simulink model "allelectronicsdraft"  (R2020a)
settings: Solver=VariableStepAuto  StartTime=0.0  StopTime=5  RelTol=1e-3
undefined symbols (not defined in the file): Ion, Lithium, sigbuilder_block
libraries: powerlib x15, electricdrivelib x13, powerlib_meascontrol x4, simulink x2, re_lib x1
settings Model: Creator=ASUS  LastModifiedBy=ASUS

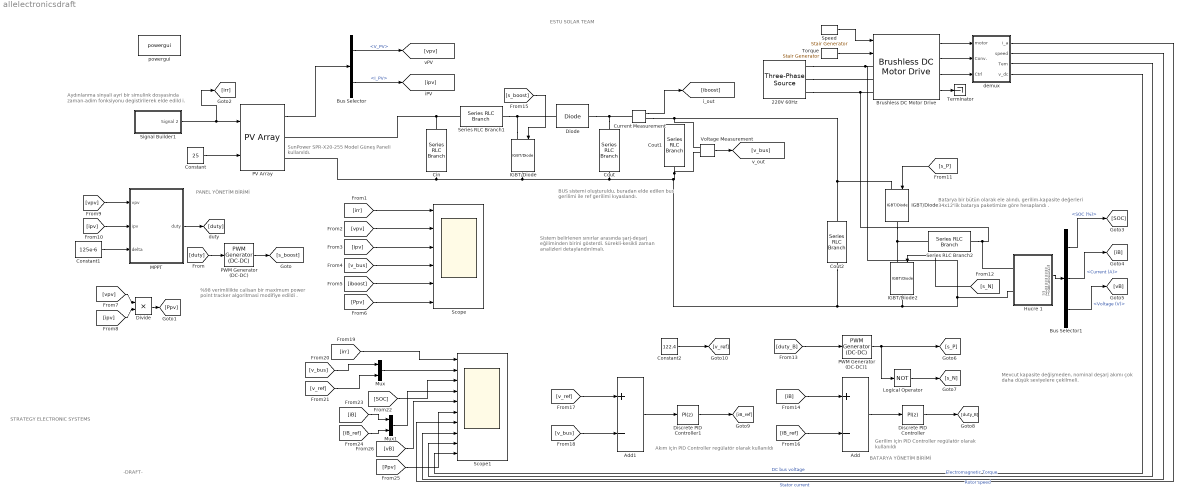
== system allelectronicsdraft ==
  note: -DRAFT-
  note: STRATEGY
      | ELECTRONIC SYSTEMS
  note: ESTU SOLAR TEAM
  note: Akım için PID Controller regülatör olarak kullanıldı
  note: PANEL YÖNETİM BİRİMİ
  note: BATARYA YÖNETİM BİRİMİ
  note: Gerilim için PID Controller regülatör olarak kullanıldı
  note: Aydınlanma sinyali ayri bir simulink dosyasinda
      | zaman-adim fonksiyonu degistirilerek elde edild i.
  note: %98 verimlilikte calisan bir maximum power
      | point tracker algoritmasi modifiye edildi .
  note: BUS sistemi oluşturuldu, buradan elde edilen
      | bus gerilimi ile ref gerilimi kıyaslandı.
  note: Batarya bir bütün olarak ele alındı, gerilim-kapasite değerleri
      | 34x12'lik batarya paketimize göre hesaplandı .
  note: Sistem belirlenen sınırlar arasında şarj-deşarj
      | eğiliminden birini gösterdi. Sürekli-kesikli zaman
      | analizleri detaylandırılmalı.
  note: Mevcut kapasite değişmeden, nominal deşarj akımı çok
      | daha düşük seviyelere çekilmeli.
  note: SunPower SPR-X20-255 Model Güneş Paneli kullanıldı.
  220V 60Hz : powerlib/Electrical Sources/Three-Phase Source  InternalConnection=Yg  VoltagePhases=off  Voltage=220  PhaseAngle=0  Voltage_phases=[25e3 25e3 25e3]/sqrt(3)  PhaseAngles_phases=[0 -120 +120]  Frequency=60  NonIdealSource=on  SpecifyImpedance=off  Resistance=0.02  Inductance=0.05e-3  ShortCircuitLevel=100e6  BaseVoltage=25e3  XRratio=7  BusType=swing  Pref=0  Qref=0  Prefabc=[10e3, 10e3, 10e3]  Qrefabc=[0, 0, 0]  Qmin=-inf  Qmax=inf
      settings: SourceProductBaseCode=MT,PS
  Add : Sum  Inputs=+-
  Add1 : Sum  Inputs=+-
  Brushless DC Motor Drive : electricdrivelib/AC drives/Brushless DC Motor Drive  Rs=0.2  Lls=8.5e-3  Flat=120  MachineConstant=Flux linkage established by magnets (V.s)  FluxCst=0.175  VoltageCst=146.6077  TorqueCst=1.4  ia=0  ib=0  J=0.089  Friction=0.005  p=4  wm=0  thetam=0  Rsnb_rec=10e3  Csnb_rec=20e-9  Ron_rec=1e-3  Vf_rec=1.3  cap_bus=2000e-6  Rbrake=8  fbrake=4000  activationVoltage=320  shutdownVoltage=310  deviceType=IGBT / Diodes  Ron_inv=1e-3  Vf_inv=0.8  Vfd_inv=0.8  Tf=1e-6  Tt=2e-6  Tf_GTO=10e-6  Tt_GTO=20e-6  Rsnb_inv=5000  Csnb_inv=inf  regulationType=Speed regulation  Acc=1000  Dec=-1000  kp_sc=3.3  ki_sc=300  fc_sc=285  Tsc=140e-6  Tmin=-17.8  Tmax=17.8  h=0.01  freq_max=20e3  Tvect=20e-6  zeta=0.99  Trd=0.13/5  K1=3000  K2=-49500  baseSampleTime=2e-06  outputBusMode=Multiple output buses  busLabels=off  sensorless=off  MechanicalLoad=Torque Tm  modelDetailLevel=Detailed  driveType=AC7  AverageValue=off
      settings: SourceProductBaseCode=PS
  Bus Selector : BusSelector  OutputSignals=V_PV,I_PV
  Bus Selector1 : BusSelector  OutputSignals=SOC (%),Current (A),Voltage (V)
  Cin : powerlib/Elements/Series RLC Branch  LConnTagsString=__new0  RConnTagsString=__new0  BranchType=RC  Resistance=1e-4  Inductance=1e-3  SetiL0=off  InitialCurrent=0  Capacitance=100e-6  Setx0=off  InitialVoltage=0  Measurements=None
  Constant : Constant  Value=25
  Constant1 : Constant  Value=125e-6
  Constant2 : Constant  Value=122.4
  Cout : powerlib/Elements/Series RLC Branch  LConnTagsString=__new0  RConnTagsString=__new0  BranchType=RC  Resistance=1e-4  Inductance=1e-3  SetiL0=off  InitialCurrent=0  Capacitance=100e-6  Setx0=off  InitialVoltage=0  Measurements=None
  Cout1 : powerlib/Elements/Series RLC Branch  LConnTagsString=__new0  RConnTagsString=__new0  BranchType=R  Resistance=20  Inductance=1e-3  SetiL0=off  InitialCurrent=0  Capacitance=100e-6  Setx0=off  InitialVoltage=0  Measurements=None
  Cout2 : powerlib/Elements/Series RLC Branch  LConnTagsString=__new0  RConnTagsString=__new0  BranchType=RC  Resistance=1e-4  Inductance=1e-3  SetiL0=off  InitialCurrent=0  Capacitance=1000e-6  Setx0=off  InitialVoltage=0  Measurements=None
  Current Measurement : powerlib/Measurements/Current Measurement  PhasorSimulation=off  OutputType=Complex  PSBequivalent=0
  Diode : powerlib/Power Electronics/Diode  Ron=0.001  Lon=0  Vf=0.8  IC=0  UseSnubber=0  Rs=500  Cs=250e-9  Measurements=off
  Discrete PID Controller : simulink/Continuous/PID Controller  Controller=PI  Form=Parallel  TimeDomain=Discrete-time  UseExternalTs=off  SampleTime=50e-6  IntegratorMethod=Forward Euler  FilterMethod=Forward Euler  ControllerParametersSource=internal  P=0.01  I=10  D=0  UseFilter=on  N=100  TunerSelectOption=Transfer Function Based (PID Tuner App)  InitialConditionSource=internal  InitialConditionForIntegrator=0  InitialConditionForFilter=0  DifferentiatorICPrevScaledInput=0  ExternalReset=none  TrackingMode=off  Kt=1  LimitOutput=on  UpperSaturationLimit=0.95  LowerSaturationLimit=0  LinearizeAsGain=off  AntiWindupMode=none  Kb=1  POutMin=[]  POutMax=[]  IOutMin=[]  IOutMax=[]  DOutMin=[]  DOutMax=[]  NOutMin=[]  NOutMax=[]  SumOutMin=[]  SumOutMax=[]  SaturationOutMin=[]  SaturationOutMax=[]  PParamMin=[]  PParamMax=[]  IParamMin=[]  IParamMax=[]  DParamMin=[]  DParamMax=[]  NParamMin=[]  NParamMax=[]  KbParamMin=[]  KbParamMax=[]  KtParamMin=[]  KtParamMax=[]  KbOutMin=[]  KbOutMax=[]  KtOutMin=[]  KtOutMax=[]  IntegratorOutMin=[]  IntegratorOutMax=[]  FilterOutMin=[]  FilterOutMax=[]  SumI1OutMin=[]  SumI1OutMax=[]  SumI2OutMin=[]  SumI2OutMax=[]  SumI3OutMin=[]  SumI3OutMax=[]  SumI4OutMin=[]  SumI4OutMax=[]  SumDOutMin=[]  SumDOutMax=[]  DifferentiatorOutMin=[]  DifferentiatorOutMax=[]  FilterDiffOutCoefMin=[]  FilterDiffOutCoefMax=[]  ReciprocalOutMin=[]  ReciprocalOutMax=[]  SumDenOutMin=[]  SumDenOutMax=[]  SumNumOutMin=[]  SumNumOutMax=[]  DivideOutMin=[]  DivideOutMax=[]  UdiffTsProdOutMin=[]  UdiffTsProdOutMax=[]  NTsProdOutMin=[]  NTsProdOutMax=[]  UintegralTsProdOutMin=[]  UintegralTsProdOutMax=[]  UngainTsProdOutMin=[]  UngainTsProdOutMax=[]  IntegratorContinuousStateAttributes=''  IntegratorStateMustResolveToSignalObject=off  IntegratorRTWStateStorageClass=Auto  FilterContinuousStateAttributes=''  FilterStateMustResolveToSignalObject=off  FilterRTWStateStorageClass=Auto  ParallelPVariant=InternalParameters  IdealPVariant=Disabled  IVariant=InternalParameters  DVariant=Disabled  IntegratorVariant=Discrete  SatVariant=Enabled  AWVariant=Passthrough  PCopyVariant=Disabled  TRVariant=Disabled  FdbkBlocksVariant=Forward  IdealPFdbkVariant=Disabled  SatFdbkVariant=Disabled  DerivativeFilterVariant=Disabled  NVariant=Disabled  NCopyVariant=Disabled_SignalSpec  FilterICVariant=Disabled  IntegratorICVariant=InternalICs  ExternalResetVariant=Disabled  TRSumVariant=Passthrough  SumFdbkVariant=Disabled  SumVariant=Sum_PI  TsampFilterVariant=InternalTs  TsampNgainVariant=Passthrough  TsampIntegralVariant=Passthrough
  Discrete PID Controller1 : simulink/Continuous/PID Controller  Controller=PI  Form=Parallel  TimeDomain=Discrete-time  UseExternalTs=off  SampleTime=500e-6  IntegratorMethod=Forward Euler  FilterMethod=Forward Euler  ControllerParametersSource=internal  P=0.85  I=10  D=0  UseFilter=on  N=100  TunerSelectOption=Transfer Function Based (PID Tuner App)  InitialConditionSource=internal  InitialConditionForIntegrator=0  InitialConditionForFilter=0  DifferentiatorICPrevScaledInput=0  ExternalReset=none  TrackingMode=off  Kt=1  LimitOutput=on  UpperSaturationLimit=50  LowerSaturationLimit=-50  LinearizeAsGain=off  AntiWindupMode=none  Kb=1  POutMin=[]  POutMax=[]  IOutMin=[]  IOutMax=[]  DOutMin=[]  DOutMax=[]  NOutMin=[]  NOutMax=[]  SumOutMin=[]  SumOutMax=[]  SaturationOutMin=[]  SaturationOutMax=[]  PParamMin=[]  PParamMax=[]  IParamMin=[]  IParamMax=[]  DParamMin=[]  DParamMax=[]  NParamMin=[]  NParamMax=[]  KbParamMin=[]  KbParamMax=[]  KtParamMin=[]  KtParamMax=[]  KbOutMin=[]  KbOutMax=[]  KtOutMin=[]  KtOutMax=[]  IntegratorOutMin=[]  IntegratorOutMax=[]  FilterOutMin=[]  FilterOutMax=[]  SumI1OutMin=[]  SumI1OutMax=[]  SumI2OutMin=[]  SumI2OutMax=[]  SumI3OutMin=[]  SumI3OutMax=[]  SumI4OutMin=[]  SumI4OutMax=[]  SumDOutMin=[]  SumDOutMax=[]  DifferentiatorOutMin=[]  DifferentiatorOutMax=[]  FilterDiffOutCoefMin=[]  FilterDiffOutCoefMax=[]  ReciprocalOutMin=[]  ReciprocalOutMax=[]  SumDenOutMin=[]  SumDenOutMax=[]  SumNumOutMin=[]  SumNumOutMax=[]  DivideOutMin=[]  DivideOutMax=[]  UdiffTsProdOutMin=[]  UdiffTsProdOutMax=[]  NTsProdOutMin=[]  NTsProdOutMax=[]  UintegralTsProdOutMin=[]  UintegralTsProdOutMax=[]  UngainTsProdOutMin=[]  UngainTsProdOutMax=[]  IntegratorContinuousStateAttributes=''  IntegratorStateMustResolveToSignalObject=off  IntegratorRTWStateStorageClass=Auto  FilterContinuousStateAttributes=''  FilterStateMustResolveToSignalObject=off  FilterRTWStateStorageClass=Auto  ParallelPVariant=InternalParameters  IdealPVariant=Disabled  IVariant=InternalParameters  DVariant=Disabled  IntegratorVariant=Discrete  SatVariant=Enabled  AWVariant=Passthrough  PCopyVariant=Disabled  TRVariant=Disabled  FdbkBlocksVariant=Forward  IdealPFdbkVariant=Disabled  SatFdbkVariant=Disabled  DerivativeFilterVariant=Disabled  NVariant=Disabled  NCopyVariant=Disabled_SignalSpec  FilterICVariant=Disabled  IntegratorICVariant=InternalICs  ExternalResetVariant=Disabled  TRSumVariant=Passthrough  SumFdbkVariant=Disabled  SumVariant=Sum_PI  TsampFilterVariant=InternalTs  TsampNgainVariant=Passthrough  TsampIntegralVariant=Passthrough
  Divide : Product  Inputs=**
  Hucre 1 : Subsystem
      mask Display: image('$imagefile'); % Use "Edit Image" on toolstrip to change.
  IGBT/Diode : powerlib/Power Electronics/IGBT//Diode  Ron=1e-3  Rs=1e5  Cs=inf  Measurements=off
  IGBT/Diode1 : powerlib/Power Electronics/IGBT//Diode  Ron=1e-3  Rs=1e5  Cs=inf  Measurements=off
  IGBT/Diode2 : powerlib/Power Electronics/IGBT//Diode  Ron=1e-3  Rs=1e5  Cs=inf  Measurements=off
  Logical Operator : Logic  Operator=NOT  AllPortsSameDT=off  OutDataTypeStr=boolean
  MPPT : MATLAB Function  TreatAsAtomicUnit=on
  Mux : Mux  Inputs=2
  Mux1 : Mux  Inputs=2
  PV Array : re_lib/Solar/PV Array  Npar=1  Nser=1  PlotType=array @ 1000 W/m2 & specified temperatures  S_vec="[ 1000  500  100 ]"  Temp_C_vec="[ 45 25  ]"  ModuleName=SunPower SPR-X20-255  PlotWhenSelected=off  Pm=254.66  Ncell=72  Voc=51  Isc=6.3  Vm=42.8  Im=5.95  beta_Voc_pc=-0.24  alpha_Isc_pc=0.04  beta_Voc=-0.1224  alpha_Isc=0.00252  IL=6.3062  I0=1.343e-12  nI=0.94549  Rsh=449.4638  Rs=0.44063  RobustModel=off  RobustCellTemperature=25  BAL=on  Tc=1e-6  Tfilter=5e-5
  PWM Generator (DC-DC) : powerlib_meascontrol/Pulse & Signal Generators/PWM Generator (DC-DC)  Fsw=5000  Ts=10e-6
  PWM Generator (DC-DC)1 : powerlib_meascontrol/Pulse & Signal Generators/PWM Generator (DC-DC)  Fsw=5000  Ts=10e-6
  Scope : Scope  NumInputPorts=6
  Scope1 : Scope  NumInputPorts=10
  Series RLC Branch1 : powerlib/Elements/Series RLC Branch  LConnTagsString=__new0  RConnTagsString=__new0  BranchType=RL  Resistance=0.1  Inductance=2e-3  SetiL0=off  InitialCurrent=0  Capacitance=100e-6  Setx0=off  InitialVoltage=0  Measurements=None
  Series RLC Branch2 : powerlib/Elements/Series RLC Branch  LConnTagsString=__new0  RConnTagsString=__new0  BranchType=RL  Resistance=0.1  Inductance=0.5e-3  SetiL0=off  InitialCurrent=0  Capacitance=100e-6  Setx0=off  InitialVoltage=0  Measurements=None
  Signal Builder1 : Subsystem  Tag=STV Subsys  LoadFcn=sigbuilder_block('load');  StartFcn=sigbuilder_block('start');  StopFcn=sigbuilder_block('stop');  ClipboardFcn=sigbuilder_block('clipboard');  mask(Sigbuilder block){tuvar=[0:10]}
      mask help: Simulink:masks:SigbuilderBlock_MD
      mask init:
      | if ~strcmp(get_param(bdroot(gcbh),'SimulationStatus'),'stopped') tuvar = sigbuilder_block('maskInit'); end
      settings: CopyFcn=sigbuilder_block('copy');  DeleteFcn=sigbuilder_block('delete');  ModelCloseFcn=sigbuilder_block('modelClose');  PreSaveFcn=sigbuilder_block('preSave');  PauseFcn=sigbuilder_block('pause');  ContinueFcn=sigbuilder_block('continue');  NameChangeFcn=sigbuilder_block('namechange');  OpenFcn=sigbuilder_block('open',[437.6 199.2 550.4 400 ]);  CloseFcn=sigbuilder_block('close');
      mask Display: plot(0, 0, 100, 100,[2, 2, 32, 32, 2], [68, 8, 8, 68, 68],[32, 2], [38, 38], [32, 19, 2],[53, 60, 44], [32, 17, 17, 2],[16, 16, 31, 31]);txt = getActiveGroup(gcbh);text(2, 100, txt,'verticalAlignment', 'top');
  Speed : powerlib_meascontrol/Pulse & Signal Generators/Stair Generator  t=[0 1]  e=[100 0]  Ts=40e-6
      settings: SourceProductBaseCode=MT,PS
  Terminator : Terminator
  Torque : powerlib_meascontrol/Pulse & Signal Generators/Stair Generator  t=[0.5 1.5]  e=[11 -11]  Ts=40e-6
      settings: SourceProductBaseCode=MT,PS
  Voltage Measurement : powerlib/Measurements/Voltage Measurement  PhasorSimulation=off  OutputType=Complex  PSBequivalent=0
  demux : Subsystem
  powergui : powerlib/powergui  Priority=1  SimulationMode=Discrete  SampleTime=2e-6  frequency=60  Iterations=50  frequencyindice=0  Pbase=100e6  ErrMax=1e-4  UnitsV=kV  UnitsW=MW  buscounter=0  FunctionMessages=off  echomessages=off  EnableUseOfTLC=off  CurrentSourceSwitches=off  DisableSnubberDevices=off  DisableRonSwitches=off  DisableVfSwitches=off  DisplayEquations=off  AutomaticDiscreteSolvers=off  SolverType=Tustin/Backward Euler (TBE)  Interpol=off  ExternalGateDelay=off  methode=off  Ts=100  x0status=blocks  SPID=on  SwTol=0  HookPort=off  NonlinearTolerance=1e-4  nMaxIteration=100  ContinueOnMaxIteration=off  RestoreLinks=warning  ResistiveCurrentMeasurement=off  Frange=[0:2:500]  Ylog=off  Xlog=on  ShowGrid=off  save=off  variable=ZData  structure=0  ZoomFFT=off  StartTime=0.0  cycles=1  DisplayStyle=1  fundamental=60  FreqAxis=off  MaxFrequency=1000  frequencyindicesteady=1  RmsSteady=1  display=off
  wires:
  [s_boost] -> IGBT/Diode/1
  Voltage Measurement/1 -> [v_bus]
  Constant/1 -> PV Array/2
  Bus Selector/2 -> [ipv]  "<I_PV>"
  Bus Selector/1 -> [vpv]  "<V_PV>"
  PV Array/1 -> Bus Selector/1
  Signal Builder1/1(Signal 2) -> [irr], PV Array/1
  Current Measurement/1 -> [iboost]
  [irr] -> Scope/1
  [vpv] -> Scope/2
  [ipv] -> Scope/3
  [v_bus] -> Scope/4
  [iboost] -> Scope/5
  [Ppv] -> Scope/6
  [vpv] -> Divide/1
  [ipv] -> Divide/2
  Divide/1 -> [Ppv]
  [duty] -> PWM Generator (DC-DC)/1
  PWM Generator (DC-DC)/1 -> [s_boost]
  MPPT/1(duty) -> [duty]
  [ipv] -> MPPT/2(ipv)
  [vpv] -> MPPT/1(vpv)
  Constant1/1 -> MPPT/3(delta)
  Bus Selector1/1 -> [SOC]  "<SOC (%)>"
  Bus Selector1/2 -> [iB]  "<Current (A)>"
  Bus Selector1/3 -> [vB]  "<Voltage (V)>"
  [s_P] -> IGBT/Diode1/1
  [s_N] -> IGBT/Diode2/1
  PWM Generator (DC-DC)1/1 -> Logical Operator/1, [s_P]
  Logical Operator/1 -> [s_N]
  [duty_B] -> PWM Generator (DC-DC)1/1
  Discrete PID Controller/1 -> [duty_B]
  Add/1 -> Discrete PID Controller/1
  [iB] -> Add/1
  [iB_ref] -> Add/2
  Discrete PID Controller1/1 -> [iB_ref]
  [v_ref] -> Add1/1
  [v_bus] -> Add1/2
  Add1/1 -> Discrete PID Controller1/1
  Constant2/1 -> [v_ref]
  [irr] -> Scope1/1
  [v_bus] -> Mux/1
  [v_ref] -> Mux/2
  [iB] -> Mux1/1
  [iB_ref] -> Mux1/2
  Brushless DC Motor Drive/4 -> Terminator/1
  demux/1(i_a) -> Scope1/7  "Stator current"
  Brushless DC Motor Drive/3 -> demux/3(Ctrl)
  Brushless DC Motor Drive/1 -> demux/1(motor)
  demux/2(speed) -> Scope1/8  "Rotor speed"
  demux/4(v_dc) -> Scope1/10  "DC bus voltage"
  Torque/1 -> Brushless DC Motor Drive/2
  demux/3(Tem) -> Scope1/9  "Electromagnetic Torque"
  Speed/1 -> Brushless DC Motor Drive/1
  Brushless DC Motor Drive/2 -> demux/2(Conv.)
  Mux/1 -> Scope1/2
  [SOC] -> Scope1/3
  Mux1/1 -> Scope1/4
  [vB] -> Scope1/5
  [Ppv] -> Scope1/6
  Hucre 1/5(m4) -> Bus Selector1/1
  connections:
  Cout/LConn1 -- Diode/RConn1 -- Current Measurement/LConn1
  PV Array/RConn1 -- Cin/LConn1 -- Series RLC Branch1/LConn1
  IGBT/Diode/LConn1 -- Series RLC Branch1/RConn1 -- Diode/LConn1
  IGBT/Diode1/RConn1 -- Series RLC Branch2/LConn1 -- IGBT/Diode2/LConn1
  Voltage Measurement/LConn1 -- Cout2/LConn1 -- IGBT/Diode1/LConn1 -- Current Measurement/RConn1
  Series RLC Branch2/RConn1 -- Hucre 1/LConn1 -- 220V 60Hz/RConn3 -- Brushless DC Motor Drive/LConn3
  PV Array/RConn2 -- Cin/RConn1 -- Cout2/RConn1 -- Hucre 1/LConn2 -- 220V 60Hz/RConn1 -- Brushless DC Motor Drive/LConn1 -- IGBT/Diode2/RConn1 -- Voltage Measurement/LConn2 -- Cout1/RConn1 -- Cout/RConn1 -- IGBT/Diode/RConn1
  220V 60Hz/RConn2 -- Brushless DC Motor Drive/LConn2

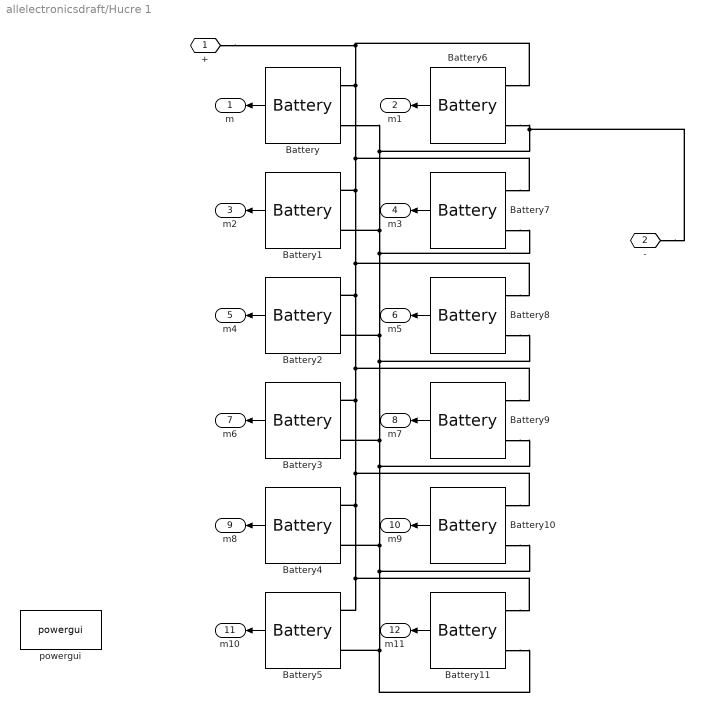
== system allelectronicsdraft/Hucre 1 ==
  Battery{,1..6,8..11} (11 alike) : electricdrivelib/Extra Sources/Battery  BatType=Lithium-Ion  ShowTempParam=off  ThermalPreset="3.6V  3.6Ah  (LiNiO2)"  ShowAgeParam=off  NomV=3.6  NomQ=3.2  SOC=95  Batt_Tr=30  PresetModel=off  MaxQ=3.35  MinV=2.5  FullV=4.2  Dis_rate=4.8  R=0.005  Normal_OP=3.25  expZone="[3.7        0.5]"  current=[6.5 13 32.5]  Units=Time  Tci=20  NomT=20  T2=0  MaxQ2=2.7  FullV2=3.5  Normal_OP2=2.94  expZone2="[3.25         0.5]"  Rca=0.6  ti=1000  Dp=0  Neq0=0  Tsim=1e6  Ta1=25  Qeol=5.4*0.9  Reol=0.013333*1.2  Char_age=[2.3478, 3]  Dis_age=[2.3478, 10]  N1=1500  N2=10500  N3=1000  N4=1400  Ta2=45  N5=950
  Battery7 : electricdrivelib/Extra Sources/Battery  BatType=Lithium-Ion  ShowTempParam=off  ThermalPreset="3.6V  3.6Ah  (LiNiO2)"  ShowAgeParam=off  NomV=3.6  NomQ=3.2  SOC=95  Batt_Tr=30  PresetModel=off  MaxQ=3.35  MinV=2.5  FullV=4.2  Dis_rate=4.8  R=0.005  Normal_OP=3.25  expZone="[3.7         0.5]"  current=[6.5 13 32.5]  Units=Time  Tci=20  NomT=20  T2=0  MaxQ2=2.7  FullV2=3.5  Normal_OP2=2.94  expZone2="[3.25         0.5]"  Rca=0.6  ti=1000  Dp=0  Neq0=0  Tsim=1e6  Ta1=25  Qeol=5.4*0.9  Reol=0.013333*1.2  Char_age=[2.3478, 3]  Dis_age=[2.3478, 10]  N1=1500  N2=10500  N3=1000  N4=1400  Ta2=45  N5=950
  powergui : powerlib/powergui  Priority=1  SimulationMode=Continuous  SampleTime=50e-6  frequency=60  Iterations=50  frequencyindice=60  Pbase=100e6  ErrMax=1e-4  UnitsV=kV  UnitsW=MW  buscounter=0  FunctionMessages=off  echomessages=off  EnableUseOfTLC=off  CurrentSourceSwitches=off  DisableSnubberDevices=off  DisableRonSwitches=off  DisableVfSwitches=off  DisplayEquations=off  AutomaticDiscreteSolvers=off  SolverType=Tustin/Backward Euler (TBE)  Interpol=off  ExternalGateDelay=off  methode=off  Ts=100  x0status=blocks  SPID=on  SwTol=0  HookPort=off  NonlinearTolerance=1e-4  nMaxIteration=100  ContinueOnMaxIteration=off  RestoreLinks=warning  ResistiveCurrentMeasurement=off  Frange=[0:2:500]  Ylog=off  Xlog=on  ShowGrid=off  save=off  variable=ZData  structure=0  ZoomFFT=off  StartTime=0.0  cycles=1  DisplayStyle=1  fundamental=60  FreqAxis=off  MaxFrequency=1000  frequencyindicesteady=1  RmsSteady=1  display=off
  + : PMIOPort  Side=Left
  - : PMIOPort  Port=2  Side=Left
  m : Outport
  m1 : Outport  Port=2
  m2 : Outport  Port=3
  m3 : Outport  Port=4
  m4 : Outport  Port=5
  m5 : Outport  Port=6
  m6 : Outport  Port=7
  m7 : Outport  Port=8
  m8 : Outport  Port=9
  m9 : Outport  Port=10
  m10 : Outport  Port=11
  m11 : Outport  Port=12
  wires:
  Battery/1 -> m/1
  Battery5/1 -> m10/1
  Battery4/1 -> m8/1
  Battery1/1 -> m2/1
  Battery2/1 -> m4/1
  Battery6/1 -> m1/1
  Battery11/1 -> m11/1
  Battery3/1 -> m6/1
  Battery10/1 -> m9/1
  Battery9/1 -> m7/1
  Battery7/1 -> m3/1
  Battery8/1 -> m5/1
  connections:
  Battery/LConn1 -- +/RConn1 -- Battery6/LConn1 -- Battery7/LConn1 -- Battery8/LConn1 -- Battery9/LConn1 -- Battery10/LConn1 -- Battery11/LConn1 -- Battery5/LConn1 -- Battery4/LConn1 -- Battery3/LConn1 -- Battery2/LConn1 -- Battery1/LConn1
  Battery/LConn2 -- -/RConn1 -- Battery6/LConn2 -- Battery7/LConn2 -- Battery8/LConn2 -- Battery3/LConn2 -- Battery9/LConn2 -- Battery4/LConn2 -- Battery10/LConn2 -- Battery11/LConn2 -- Battery5/LConn2 -- Battery2/LConn2 -- Battery1/LConn2

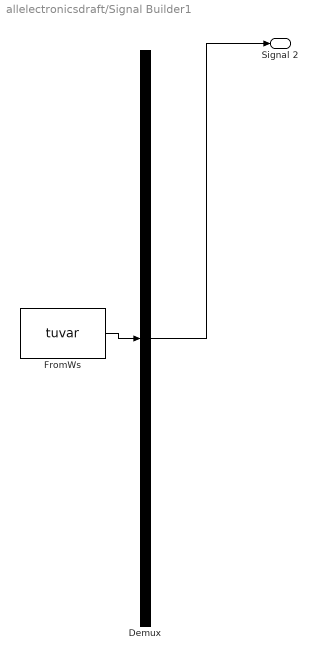
== system allelectronicsdraft/Signal Builder1 ==
  Demux : Demux  Tag=STV Demux  Outputs=1
      settings: DisplayOption=none
  FromWs : FromWorkspace  Tag=STV FromWs  VariableName=tuvar
      SigBuilderData=|
      | common.afterFinalStr = 'Extrapolate'
      | common.sampleTime = 0
      | dataSet.timeRange = [0 30]
      | dataSet.name = 'Group 1'
      | sbobj.Groups.Name = 'Group 1'
      | sbobj.Groups.Signals.Name = 'Signal 2'
      | sbobj.Groups.Signals.XData = [0 0.0312174817898 0.0624349635796 0.0936524453694 0.124869927159 0.156087408949 0.187304890739 0.218522372529 0.249739854318 0.280957336108 0.312174817898 0.343392299688 ... (962 elements, 1x962)]
      | sbobj.Groups.Signals.YData = [2.37993 2.37993 2.37993 2.37993 2.37993 2.37993 2.37993 2.37993 2.37993 2.37992 2.37992 2.37992 ... (962 elements, 1x962)]
      | sbobj.Groups.TimeRange = [0 30]
  Signal 2 : Outport  Tag=STV Outport
  wires:
  FromWs/1 -> Demux/1
  Demux/1 -> Signal 2/1

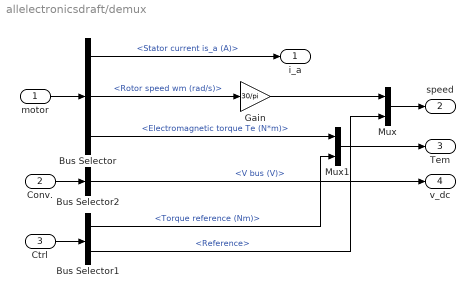
== system allelectronicsdraft/demux ==
  motor : Inport
  Conv. : Inport  Port=2
  Ctrl : Inport  Port=3
  Bus Selector : BusSelector  OutputSignals=Stator current is_a (A),Rotor speed wm (rad/s),Electromagnetic torque Te (N*m)
  Bus Selector1 : BusSelector  OutputSignals=Torque reference (Nm),Reference
  Bus Selector2 : BusSelector  OutputSignals=V bus (V)
  Gain : Gain  Gain=30/pi  SaturateOnIntegerOverflow=on  OutDataTypeStr=Inherit: Same as input  ParamDataTypeStr=Inherit: Same as input
  Mux : Mux  Inputs=2
  Mux1 : Mux  Inputs=2
  i_a : Outport  VectorParamsAs1DForOutWhenUnconnected=off
  speed : Outport  Port=2  VectorParamsAs1DForOutWhenUnconnected=off
  Tem : Outport  Port=3  VectorParamsAs1DForOutWhenUnconnected=off
  v_dc : Outport  Port=4  VectorParamsAs1DForOutWhenUnconnected=off
  wires:
  Bus Selector/2 -> Gain/1  "<Rotor speed wm (rad/s)>"
  Bus Selector2/1 -> v_dc/1  "<V bus (V)>"
  Conv./1 -> Bus Selector2/1
  Ctrl/1 -> Bus Selector1/1
  Bus Selector1/1 -> Mux1/2  "<Torque reference (Nm)>"
  Bus Selector1/2 -> Mux/2  "<Reference>"
  Gain/1 -> Mux/1
  Bus Selector/1 -> i_a/1  "<Stator current is_a (A)>"
  Bus Selector/3 -> Mux1/1  "<Electromagnetic torque Te (N*m)>"
  Mux1/1 -> Tem/1
  Mux/1 -> speed/1
  motor/1 -> Bus Selector/1

== matlab function allelectronicsdraft/MPPT ==
  data: vpv input; duty output; ipv input; delta input
function duty = MPPT_algorithm(vpv,ipv,delta)
duty_init = 0.1;
%duty limitlemesi gerceklestirildi
duty_min=0;
duty_max=0.85;
persistent Vold Pold duty_old;
%veri depolanmasi icin
if isempty(Vold)
    Vold=0;
    Pold=0;
    duty_old=duty_init;
end
P= vpv*ipv; %guc
dV=vpv-Vold; %gerilim degisimi
dP=P-Pold; %guc degisimi
if dP ~= 0 && vpv>30
    if dP<0
        if dV<0
            duty=duty_old - delta;
        else
            duty=duty_old + delta;
        end
    else
        if dV<0
            duty=duty_old + delta;
        else
            duty=duty_old - delta;
        end
    end
else
    duty=duty_old;
end
if duty >= duty_max
    duty=duty_max;
elseif duty<duty_min
    duty=duty_min;
end
duty_old=duty;
Vold=vpv;
Pold=P;
